simulink model "motorDistSenSim"  (R2023a)
settings: Solver=VariableStepAuto  StartTime=0.0  StopTime=tFinal  RelTol=1e-3
values from neighbouring files (symbols this model uses):
  Jm = 10.3E-7    (= 1.03e-06)    [C7_1_motorModel.m]    (also in C7_3_motorDistSensitivity.m = 0.001)
  Km = 23.2E-3    (= 0.0232)    [C7_1_motorModel.m]    (also in C7_3_motorDistSensitivity.m = 0.2)
  Kv = 5    [C7_3_motorDistSensitivity.m]
  Kw = (Km^2 + Km*Kv)/Km    (= 5.2)    [C7_3_motorDistSensitivity.m]
  Rm = 2.32    [C7_1_motorModel.m]    (also in C7_3_motorDistSensitivity.m = 20)
  t_Td = 5    [C7_3_motorDistSensitivity.m]
  Td = 0    [C7_1_motorModel.m]    (also in C7_3_motorDistSensitivity.m = 0.01)
settings Model: Creator=jwil0  LastModifiedBy=USER
settings DebuggingCC: UnconnectedInputMsg=warning  UnconnectedOutputMsg=warning  UnconnectedLineMsg=warning
settings ModelReferenceCC: EnableRefExpFcnMdlSchedulingChecks=on
settings RTWCC: DLArmComputeVersion=19.05

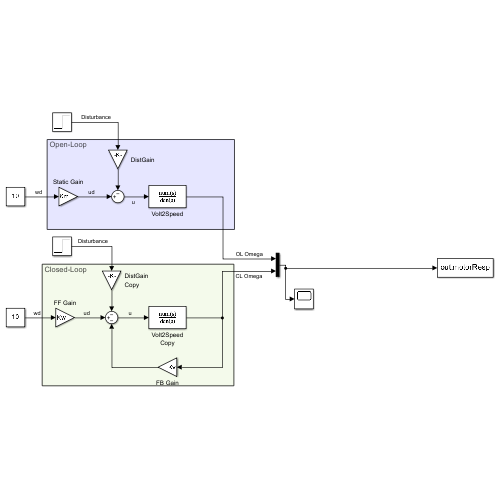
[thumbnail: Simulink's stored preview of the top-level diagram]
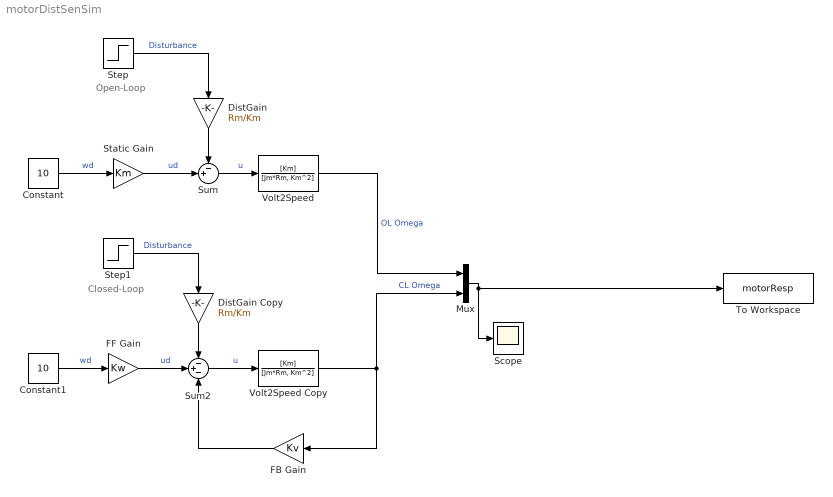
== system motorDistSenSim ==
  note: Closed-Loop
  note: Open-Loop
  Constant : Constant  Value=10
  Constant1 : Constant  Value=10
  DistGain : Gain  Gain=Rm/Km
  DistGain Copy : Gain  Gain=Rm/Km
  FB Gain : Gain  Gain=Kv
  FF Gain : Gain  Gain=Kw
  Mux : Mux  Inputs=2
  Scope : Scope
  Static Gain : Gain  Gain=Km
  Step : Step  Time=t_Td  After=Td  SampleTime=0
  Step1 : Step  Time=t_Td  After=Td  SampleTime=0
  Sum : Sum  Inputs=-+|
  Sum2 : Sum  Inputs=-+-
  To Workspace : ToWorkspace  VariableName=motorResp  SaveFormat=Timeseries  SampleTime=-1
  Volt2Speed : TransferFcn  Numerator=[Km]  Denominator=[Jm*Rm, Km^2]
  Volt2Speed Copy : TransferFcn  Numerator=[Km]  Denominator=[Jm*Rm, Km^2]
  wires:
  Volt2Speed Copy/1 -> Mux/2, FB Gain/1  "CL Omega"
  Sum2/1 -> Volt2Speed Copy/1  "u"
  FB Gain/1 -> Sum2/3
  Sum/1 -> Volt2Speed/1  "u"
  Constant/1 -> Static Gain/1  "wd"
  DistGain/1 -> Sum/1
  DistGain Copy/1 -> Sum2/1
  Step/1 -> DistGain/1  "Disturbance"
  Step1/1 -> DistGain Copy/1  "Disturbance"
  Volt2Speed/1 -> Mux/1  "OL Omega"
  FF Gain/1 -> Sum2/2  "ud"
  Constant1/1 -> FF Gain/1  "wd"
  Static Gain/1 -> Sum/2  "ud"
  Mux/1 -> Scope/1, To Workspace/1
